simulink model "RechtenMotor_2_4_simu"  (R2012b)
settings: Solver=FixedStepDiscrete  StartTime=0.0  StopTime=10.0  RelTol=1e-3
undefined symbols (not defined in the file): sigbuilder_block
libraries: c2833xlib x1, c280xlib x1
settings Model: Creator=mit064  LastModifiedBy=Gelin Wang
settings DataIOCC: SaveOutput=off  SaveTime=off
settings OptimizationCC: OptimizeModelRefInitCode=on  LifeSpan=1
settings HardwareCC: ProdBitPerChar=16  ProdBitPerInt=16  ProdBitPerPointer=16  ProdLargestAtomicInteger=Integer  ProdIntDivRoundTo=Zero  ProdEndianess=LittleEndian  ProdWordSize=16  ProdHWDeviceType=Texas Instruments->C2000
settings RTWCC: SystemTargetFile=idelink_ert.tlc  GenerateMakefile=off  TemplateMakefile=none  Description=IDE Link ERT  ProcessScript=idelink_ert_make_rtw_hook
settings CodeAppCC: IgnoreCustomStorageClasses=off

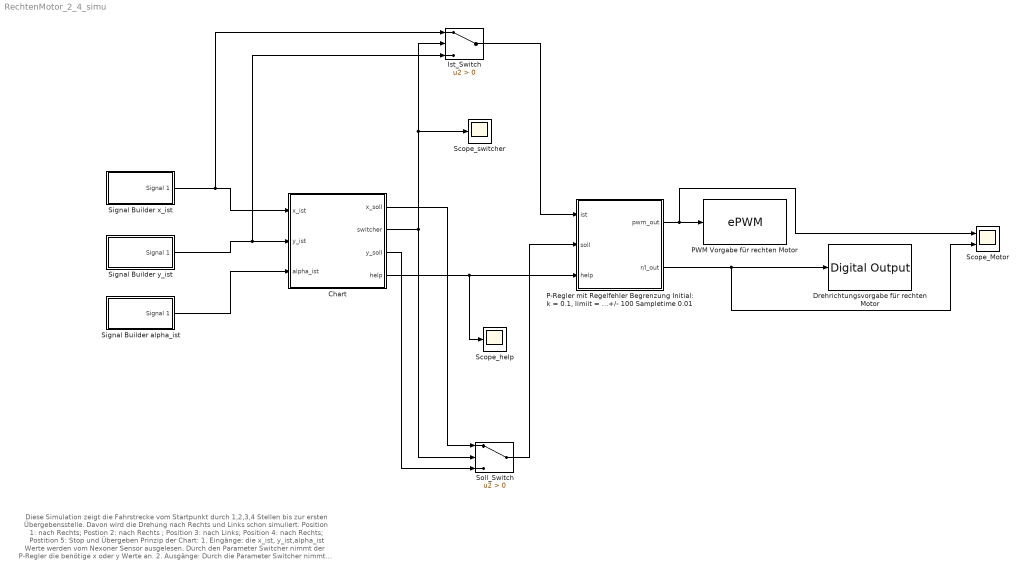
== system RechtenMotor_2_4_simu ==
  note: Diese Simulation zeigt die Fahrstrecke vom Startpunkt durch 1,2,3,4 Stellen bis zur ersten Übergebensstelle.
      | Davon wird die Drehung nach Rechts und Links schon simuliert.
      | Position 1: nach Rechts; Postion 2: nach Rechts ; Position 3: nach Links; Position 4: nach Rechts; Postition 5: Stop und Übergeben
      |
      | Prinzip der Chart:
      | 1. Eingänge: die x_ist, y_ist,alpha_ist Werte werden vom Nexoner Sensor ausgelesen.
      | Durch den Parameter Switcher nimmt der P-Regler die benötige x oder y Werte an.
      | 2. Ausgänge: Durch die Parameter Switcher nimmt ebenfalls der P-Regler die benötige x oder y Werte an.
      | 3. Parameter help in Ausgang: im Fall wenn der Fahrzeug sich nach Rechts umdrehen will, und  y_soll oder x_soll werte kleiner als den letzen Stelle ist,
      | wird "help" gleich eins, somit dreht sich der Rechtsmotor in negative Richtung .
      | 4. Parameter help in P-Regler: wenn help gleich eins ist, wird der Motor sich  immer in eine Richtung drehen.
  Chart : Stateflow chart  TreatAsAtomicUnit=on
  Drehrichtungsvorgabe für rechten Motor : c2833xlib/Digital Output  GPIO_Number=GPIO16~GPIO23  GPIO_Bit0=off  GPIO_BIT0_Toggle=off  GPIO_Bit1=off  GPIO_BIT1_Toggle=off  GPIO_Bit2=off  GPIO_BIT2_Toggle=off  GPIO_Bit3=off  GPIO_BIT3_Toggle=off  GPIO_Bit4=off  GPIO_BIT4_Toggle=off  GPIO_Bit5=on  GPIO_BIT5_Toggle=off  GPIO_Bit6=off  GPIO_BIT6_Toggle=off  GPIO_Bit7=off  GPIO_BIT7_Toggle=off
  Ist_Switch : Switch  Criteria=u2 > Threshold
  "P-Regler mit Regelfehler Begrenzung Initial: k = 0.1, limiit = +/- 100 Sampletime 0.01" : Subsystem
  "PWM Vorgabe für rechten Motor " : c280xlib/ePWM  checkMode=off  useModule=ePWM2  periodUnits=Clock cycles  timerSource=Specify via dialog  timerPeriod_clk=64000  timerPeriod_sec=0.0001  countingMode=Up  synchronizationOption=Disable  synchronizationEnable=off  phaseActiveEnable=Disable  phaseDirection=Count down after sync  phaseActive=0  clockPrescale=1  HSclockPrescale=1  ePWMxAStatus=off  CMPAUnits=Clock cycles  CMPASource=Specify via dialog  CMPAValue_per=50  CMPAValue_clk=32000  ePWMxAactionLogic1=Do nothing  ePWMxAactionLogic2=Clear  ePWMxAactionLogic3=Set  ePWMxAactionLogic4=Do nothing  ePWMxAactionLogic5=Do nothing  ePWMxAactionLogic6=Do nothing  ePWMxALoadMode=Load on CTR=Zero  ePWMxACSFenable=off  ePWMxACSFvalue=Forcing Disable  ePWMxASFreload=Zero  enHRPWM=off  HRPWM_LoadMode=CTR=ZERO  HRPWM_CTLMode=Phase control mode  HRPWM_EDGMode=Both edge  enSFO=on  ePWMxBStatus=on  CMPBUnits=Percentages  CMPBSource=Input port  CMPBValue_per=0  CMPBValue_clk=32000  ePWMxBactionLogic1=Do nothing  ePWMxBactionLogic2=Set  ePWMxBactionLogic3=Do nothing  ePWMxBactionLogic4=Do nothing  ePWMxBactionLogic5=Clear  ePWMxBactionLogic6=Do nothing  ePWMxBLoadMode=Load on CTR=Zero  ePWMxBCSFenable=off  ePWMxBCSFvalue=Forcing Disable  ePWMxBSFreload=Zero  enableDBePWMxA=off  enableDBePWMxB=off  DBpolarity=AH  DBedgeDelay=Positive  DBSource_ePWMxA=ePWMxA  DBSource_ePWMxB=ePWMxA  DBperiodSource=Specify via dialog  REDperiod=0  FEDperiod=0  adcstartModuleA=off  adcrequestEventA=First event  adcstartEventA=CTR=Zero  adcstartModuleB=off  adcrequestEventB=First event  adcstartEventB=CTR=Zero  intEn=off  intPrd=First event  intSel=CTR=Zero  chopperEnable=off  chopperFrequency=1  chopperFirstwidth=1  chopperDuty=12.5%  tripZonesource=Specify via dialog  tzselOSHT1=off  tzselOSHT2=off  tzselOSHT3=off  tzselOSHT4=off  tzselOSHT5=off  tzselOSHT6=off  tzselCBC1=off  tzselCBC2=off  tzselCBC3=off  tzselCBC4=off  tzselCBC5=off  tzselCBC6=off  enTzOstIntr=off  enTzCbcIntr=off  ePWMxAforced=No action  ePWMxBforced=No action  timerPeriod=-1  ePWMxAValue=0  ePWMxBValue=0  tripZoneoption=OSHT
  Scope_Motor : Scope  NumInputPorts=2
      settings: YMin=-5~-5  YMax=120~5
  Scope_help : Scope
      settings: SaveName=ScopeData2
  "Scope_switcher " : Scope
  "Signal Builder alpha_ist " : Subsystem  Tag=STV Subsys  LoadFcn=sigbuilder_block('load');  StartFcn=sigbuilder_block('start');  StopFcn=sigbuilder_block('stop');  ClipboardFcn=sigbuilder_block('clipboard');  mask(Sigbuilder block){}
      mask help: Simulink:masks:SigbuilderBlock_MD
      mask init:
      | if ~strcmp(get_param(bdroot(gcbh),'SimulationStatus'),'stopped') tuvar = sigbuilder_block('maskInit'); end
      settings: CopyFcn=sigbuilder_block('copy');  DeleteFcn=sigbuilder_block('delete');  ModelCloseFcn=sigbuilder_block('modelClose');  PreSaveFcn=sigbuilder_block('preSave');  PauseFcn=sigbuilder_block('pause');  ContinueFcn=sigbuilder_block('continue');  NameChangeFcn=sigbuilder_block('namechange');  OpenFcn=sigbuilder_block('open',[803.25 -542.25 550.5 399.75 ]);  CloseFcn=sigbuilder_block('close');
      mask Display: plot(0, 0, 100, 100,[2, 2, 32, 32, 2], [68, 8, 8, 68, 68],[32, 2], [38, 38], [32, 19, 2],[53, 60, 44], [32, 17, 17, 2],[16, 16, 31, 31]);txt = getActiveGroup(gcbh);text(2, 100, txt,'verticalAlignment', 'top');
  "Signal Builder x_ist " : Subsystem  Tag=STV Subsys  LoadFcn=sigbuilder_block('load');  StartFcn=sigbuilder_block('start');  StopFcn=sigbuilder_block('stop');  ClipboardFcn=sigbuilder_block('clipboard');  mask(Sigbuilder block){}
      mask help: Simulink:masks:SigbuilderBlock_MD
      mask init:
      | if ~strcmp(get_param(bdroot(gcbh),'SimulationStatus'),'stopped') tuvar = sigbuilder_block('maskInit'); end
      settings: CopyFcn=sigbuilder_block('copy');  DeleteFcn=sigbuilder_block('delete');  ModelCloseFcn=sigbuilder_block('modelClose');  PreSaveFcn=sigbuilder_block('preSave');  PauseFcn=sigbuilder_block('pause');  ContinueFcn=sigbuilder_block('continue');  NameChangeFcn=sigbuilder_block('namechange');  OpenFcn=sigbuilder_block('open',[403.5 2.25 550.5 399.75 ]);  CloseFcn=sigbuilder_block('close');
      mask Display: plot(0, 0, 100, 100,[2, 2, 32, 32, 2], [68, 8, 8, 68, 68],[32, 2], [38, 38], [32, 19, 2],[53, 60, 44], [32, 17, 17, 2],[16, 16, 31, 31]);txt = getActiveGroup(gcbh);text(2, 100, txt,'verticalAlignment', 'top');
  "Signal Builder y_ist " : Subsystem  Tag=STV Subsys  LoadFcn=sigbuilder_block('load');  StartFcn=sigbuilder_block('start');  StopFcn=sigbuilder_block('stop');  ClipboardFcn=sigbuilder_block('clipboard');  mask(Sigbuilder block){}
      mask help: Simulink:masks:SigbuilderBlock_MD
      mask init:
      | if ~strcmp(get_param(bdroot(gcbh),'SimulationStatus'),'stopped') tuvar = sigbuilder_block('maskInit'); end
      settings: CopyFcn=sigbuilder_block('copy');  DeleteFcn=sigbuilder_block('delete');  ModelCloseFcn=sigbuilder_block('modelClose');  PreSaveFcn=sigbuilder_block('preSave');  PauseFcn=sigbuilder_block('pause');  ContinueFcn=sigbuilder_block('continue');  NameChangeFcn=sigbuilder_block('namechange');  OpenFcn=sigbuilder_block('open',[1200.75 -1.5 550.5 399.75 ]);  CloseFcn=sigbuilder_block('close');
      mask Display: plot(0, 0, 100, 100,[2, 2, 32, 32, 2], [68, 8, 8, 68, 68],[32, 2], [38, 38], [32, 19, 2],[53, 60, 44], [32, 17, 17, 2],[16, 16, 31, 31]);txt = getActiveGroup(gcbh);text(2, 100, txt,'verticalAlignment', 'top');
  Soll_Switch : Switch  Criteria=u2 > Threshold
  wires:
  "P-Regler mit Regelfehler Begrenzung Initial: k = 0.1, limiit = +/- 100 Sampletime 0.01"/2(r/l_out) -> Scope_Motor/2, Drehrichtungsvorgabe für rechten Motor/1
  "P-Regler mit Regelfehler Begrenzung Initial: k = 0.1, limiit = +/- 100 Sampletime 0.01"/1(pwm_out) -> Scope_Motor/1, "PWM Vorgabe für rechten Motor "/1
  Ist_Switch/1 -> "P-Regler mit Regelfehler Begrenzung Initial: k = 0.1, limiit = +/- 100 Sampletime 0.01"/1(ist)
  Soll_Switch/1 -> "P-Regler mit Regelfehler Begrenzung Initial: k = 0.1, limiit = +/- 100 Sampletime 0.01"/2(soll)
  Chart/2(switcher) -> "Scope_switcher "/1, Ist_Switch/2, Soll_Switch/2
  Chart/1(x_soll) -> Soll_Switch/1
  Chart/3(y_soll) -> Soll_Switch/3
  Chart/4(help) -> Scope_help/1, "P-Regler mit Regelfehler Begrenzung Initial: k = 0.1, limiit = +/- 100 Sampletime 0.01"/3(help)
  "Signal Builder x_ist "/1(Signal 1) -> Ist_Switch/1, Chart/1(x_ist)
  "Signal Builder y_ist "/1(Signal 1) -> Ist_Switch/3, Chart/2(y_ist)
  "Signal Builder alpha_ist "/1(Signal 1) -> Chart/3(alpha_ist)

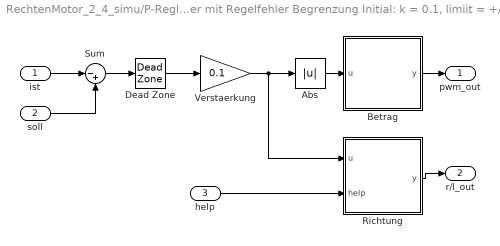
== system RechtenMotor_2_4_simu/P-Regler mit Regelfehler Begrenzung Initial: k = 0.1, limiit = +//- 100 Sampletime 0.01 ==
  ist : Inport
  soll : Inport  Port=2
  help : Inport  Port=3
  Abs : Abs  SampleTime=0.01
  Betrag : MATLAB Function  TreatAsAtomicUnit=on  SystemSampleTime=0.01
  Dead Zone : DeadZone  LowerValue=-100  UpperValue=100  SampleTime=0.01  SaturateOnIntegerOverflow=on
  Richtung : MATLAB Function  TreatAsAtomicUnit=on  SystemSampleTime=0.01
  Sum : Sum  Inputs=|-+  SampleTime=0.01
  Verstaerkung : Gain  Gain=0.1  SampleTime=0.01
  pwm_out : Outport
  r/l_out : Outport  Port=2
  wires:
  Betrag/1(y) -> pwm_out/1
  Sum/1 -> Dead Zone/1
  Verstaerkung/1 -> Abs/1, Richtung/1(u)
  Dead Zone/1 -> Verstaerkung/1
  Abs/1 -> Betrag/1(u)
  soll/1 -> Sum/2
  Richtung/1(y) -> r/l_out/1
  ist/1 -> Sum/1
  help/1 -> Richtung/2(help)

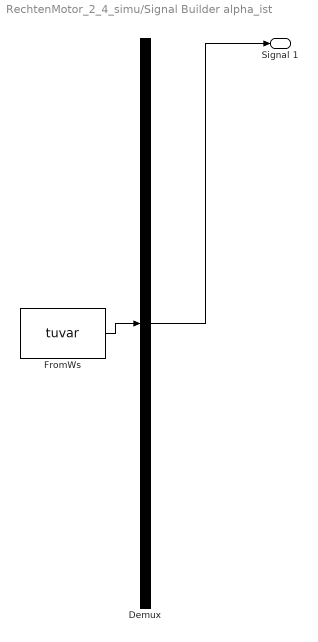
== system RechtenMotor_2_4_simu/Signal Builder alpha_ist  ==
  Demux : Demux  Tag=STV Demux  Outputs=1
  FromWs : FromWorkspace  Tag=STV FromWs  VariableName=tuvar  SampleTime=0
      SigBuilderData=|
      | common.afterFinalStr = 'Extrapolate'
      | common.sampleTime = 0
      | dataSet.timeRange = [0 25]
      | dataSet.name = 'Group 1'
      | sbobj.Groups.Name = 'Group 1'
      | sbobj.Groups.Signals.Name = 'Signal 1'
      | sbobj.Groups.Signals.XData = [0 4 5 6 9.5 10.5 14 15 18.5 19.5 25]
      | sbobj.Groups.Signals.YData = [90 90 90 77 77 -59 -59 63 63 -63 -63]
      | sbobj.Groups.TimeRange = [0 25]
  Signal 1 : Outport  Tag=STV Outport
  wires:
  Demux/1 -> Signal 1/1
  FromWs/1 -> Demux/1

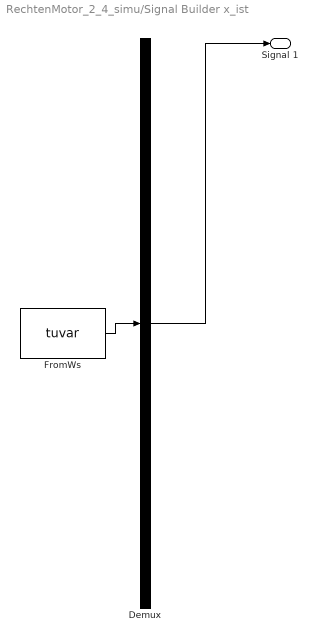
== system RechtenMotor_2_4_simu/Signal Builder x_ist  ==
  Demux : Demux  Tag=STV Demux  Outputs=1
  FromWs : FromWorkspace  Tag=STV FromWs  VariableName=tuvar  SampleTime=0
      SigBuilderData=|
      | common.afterFinalStr = 'Extrapolate'
      | common.sampleTime = 0
      | dataSet.timeRange = [0 25]
      | dataSet.name = 'Group 1'
      | sbobj.Groups.Name = 'Group 1'
      | sbobj.Groups.Signals.Name = 'Signal 1'
      | sbobj.Groups.Signals.XData = [0 4 6 6.5 8.5 11 13 15.5 17.5 20 22 25]
      | sbobj.Groups.Signals.YData = [350 350 350 350 500 500 800 800 950 950 1100 1100]
      | sbobj.Groups.TimeRange = [0 25]
  Signal 1 : Outport  Tag=STV Outport
  wires:
  Demux/1 -> Signal 1/1
  FromWs/1 -> Demux/1

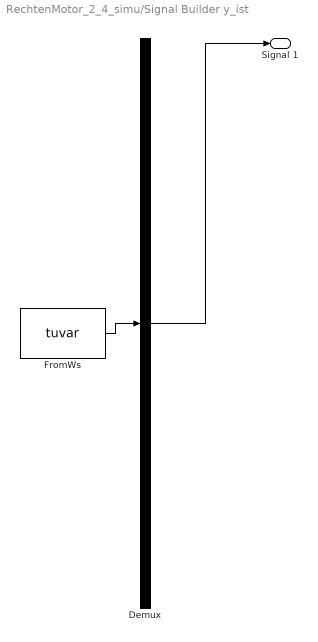
== system RechtenMotor_2_4_simu/Signal Builder y_ist  ==
  Demux : Demux  Tag=STV Demux  Outputs=1
  FromWs : FromWorkspace  Tag=STV FromWs  VariableName=tuvar  SampleTime=0
      SigBuilderData=|
      | common.afterFinalStr = 'Extrapolate'
      | common.sampleTime = 0
      | dataSet.timeRange = [0 25]
      | dataSet.name = 'Group 1'
      | sbobj.Groups.Name = 'Group 1'
      | sbobj.Groups.Signals.Name = 'Signal 1'
      | sbobj.Groups.Signals.XData = [0 2 4 6 6.5 8.5 11 13 15.5 17.5 20 22 25]
      | sbobj.Groups.Signals.YData = [0 0 250 250 250 900 900 400 400 700 700 400 400]
      | sbobj.Groups.TimeRange = [0 25]
  Signal 1 : Outport  Tag=STV Outport
  wires:
  Demux/1 -> Signal 1/1
  FromWs/1 -> Demux/1

== stateflow chart RechtenMotor_2_4_simu/Chart ==
  state Start
  state Position_3
    exit:switcher=0;
    exit:help=1;
    state Position_2
      entry:y_soll=400;
    state Stop
      entry:y_soll=y_ist;
    state Drehen_Linke
      entry:y_soll=0;
    state stop
      entry:y_soll=y_ist;
    (default) -> Position_3.Position_2
    Position_3.Position_2 -> Position_3.Stop : [y_ist<402&&y_ist>398]
    Position_3.Stop -> Position_3.Drehen_Linke : [after(1,sec)]
    Position_3.Drehen_Linke -> Position_3.stop : [alpha_ist<65&&alpha_ist>61]
  state Position_4
    exit:switcher=0;
    exit:help=0;
    state Position_3
      entry:y_soll=700;
    state Stop
      entry:y_soll=y_ist;
    state Drehen_Recht
      entry:y_soll=0;
    state stop
      entry:y_soll=y_ist;
    (default) -> Position_4.Position_3
    Position_4.Position_3 -> Position_4.Stop : [y_ist<702&&y_ist>698]
    Position_4.Stop -> Position_4.Drehen_Recht : [after(1,sec)]
    Position_4.Drehen_Recht -> Position_4.stop : [alpha_ist<-61&&alpha_ist>-65]
  state Position_1
    exit:switcher=0;
    exit:help=0;
    state Position_1
      entry:y_soll=350;
    state Stop
      entry:y_soll=y_ist;
    state Drehen_Recht
      entry:y_soll=0;
    state stop
      entry:y_soll=y_ist;
    (default) -> Position_1.Position_1
    Position_1.Position_1 -> Position_1.Stop : [y_ist<352&&y_ist>348]
    Position_1.Stop -> Position_1.Drehen_Recht : [after(1,sec)]
    Position_1.Drehen_Recht -> Position_1.stop : [alpha_ist<79&&alpha_ist>75]
  state Position_2
    exit:switcher=0;
    exit:help=0;
    state Position_2
      entry:y_soll=900;
    state Stop
      entry:y_soll=y_ist;
    state Drehen_Recht
      entry:y_soll=0;
    state stop
      entry:y_soll=y_ist;
    (default) -> Position_2.Position_2
    Position_2.Position_2 -> Position_2.Stop : [y_ist<902&&y_ist>898]
    Position_2.Stop -> Position_2.Drehen_Recht : [after(1,sec)]
    Position_2.Drehen_Recht -> Position_2.stop : [alpha_ist>-61&&alpha_ist<-57]
  state Position_6
    exit:switcher=0;
    exit:help=1;
    state Position_2
      entry:y_soll=300;
    state Stop
      entry:y_soll=y_ist;
    state Drehen_Linke
      entry:y_soll=0;
    state stop
      entry:y_soll=y_ist;
    (default) -> Position_6.Position_2
    Position_6.Position_2 -> Position_6.Stop : [y_ist<302&&y_ist>298]
    Position_6.Stop -> Position_6.Drehen_Linke : [after(1,sec)]
    Position_6.Drehen_Linke -> Position_6.stop : [alpha_ist<-32&&alpha_ist>-36]
  state Position_5_give
    exit:switcher=0;
    exit:help=0;
    state Position_1
      entry:y_soll=400;
    state Stop
      entry:y_soll=y_ist;
    state Drehen_Recht
      entry:y_soll=0;
    state stop
      entry:y_soll=y_ist;
    (default) -> Position_5_give.Position_1
    Position_5_give.Position_1 -> Position_5_give.Stop : [y_ist<402&&y_ist>398]
    Position_5_give.Stop -> Position_5_give.Drehen_Recht : [after(5,sec)]
    Position_5_give.Drehen_Recht -> Position_5_give.stop : [alpha_ist<-88]
  state Position_7
    exit:switcher=1;
    exit:help=1;
    state Position_2
      entry:x_soll=1400;
    state Stop
      entry:x_soll=x_ist;
    state Drehen_Linke
      entry:x_soll=0;
    state stop
      entry:x_soll=x_ist;
    (default) -> Position_7.Position_2
    Position_7.Position_2 -> Position_7.Stop : [x_ist<1402&&x_ist>1398]
    Position_7.Stop -> Position_7.Drehen_Linke : [after(1,sec)]
    Position_7.Drehen_Linke -> Position_7.stop : [alpha_ist<47&&alpha_ist>43]
  state Position_8
    exit:switcher=1;
    exit:help=1;
    state Position_2
      entry:x_soll=1700;
    state Stop
      entry:x_soll=x_ist;
    state Drehen_Linke
      entry:x_soll=0;
    state stop
      entry:x_soll=x_ist;
    (default) -> Position_8.Position_2
    Position_8.Position_2 -> Position_8.Stop : [x_ist<1702&&x_ist>1698]
    Position_8.Stop -> Position_8.Drehen_Linke : [after(1,sec)]
    Position_8.Drehen_Linke -> Position_8.stop : [alpha_ist<47&&alpha_ist>43]
  state Position_11_give
    exit:switcher=0;
    exit:help=1;
    state Position_2
      entry:y_soll=300;
    state Stop
      entry:y_soll=y_ist;
    (default) -> Position_11_give.Position_2
    Position_11_give.Position_2 -> Position_11_give.Stop : [y_ist<302&&y_ist>298]
  state Position_12_End
    exit:switcher=0;
    exit:help=1;
    state Position_2
      entry:y_soll=-200;
    state Stop
      entry:y_soll=y_ist;
    (default) -> Position_12_End.Position_2
    Position_12_End.Position_2 -> Position_12_End.Stop : [y_ist<-198&&y_ist>-202]
  state Position_9
    exit:switcher=1;
    exit:help=1;
    state Position_2
      entry:x_soll=1100;
    state Stop
      entry:x_soll=x_ist;
    state Drehen_Linke
      entry:x_soll=0;
    state stop
      entry:x_soll=x_ist;
    (default) -> Position_9.Position_2
    Position_9.Position_2 -> Position_9.Stop : [x_ist<1102&&x_ist>1098]
    Position_9.Stop -> Position_9.Drehen_Linke : [after(1,sec)]
    Position_9.Drehen_Linke -> Position_9.stop : [alpha_ist<2&&alpha_ist>-2]
  state Position_10
    exit:switcher=0;
    exit:help=1;
    state Position_2
      entry:y_soll=300;
    state Stop
      entry:y_soll=y_ist;
    state Drehen_Linke
      entry:y_soll=0;
    state stop
      entry:y_soll=y_ist;
    (default) -> Position_10.Position_2
    Position_10.Position_2 -> Position_10.Stop : [y_ist<302&&y_ist>298]
    Position_10.Stop -> Position_10.Drehen_Linke : [after(1,sec)]
    Position_10.Drehen_Linke -> Position_10.stop : [alpha_ist<-88]
  (default) -> Start
  Start -> Position_1 : [after(2,sec)]
  Position_3 -> Position_4 : [after(0.5,sec)]
  Position_1 -> Position_2 : [after(0.5,sec)]
  Position_2 -> Position_3 : [after(0.5,sec)]
  Position_4 -> Position_5_give : [after(0.5,sec)]
  Position_7 -> Position_8 : [after(0.5,sec)]
  Position_6 -> Position_7 : [after(0.5,sec)]
  Position_5_give -> Position_6 : [after(0.5,sec)]
  Position_8 -> Position_9 : [after(0.5,sec)]
  Position_11_give -> Position_12_End : [after(5,sec)]
  Position_9 -> Position_10 : [after(0.5,sec)]
  Position_10 -> Position_11_give : [after(0.5,sec)]
  data: x_ist input; y_ist input; alpha_ist input; x_soll output; switcher output; y_soll output; help output

== matlab function RechtenMotor_2_4_simu/P-Regler mit Regelfehler Begrenzung Initial: k = 0.1, limiit = +//- 100 Sampletime 0.01/Betrag ==
  settings: updateMethod=DISCRETE  sampleTime=0.01
  data: u input; y output
function y = fcn( u )

if 0.5 < u && u < 60
    y = 60;
elseif u <= 0.5
    y = 0;
elseif u >= 100
    y = 100;
else
    y = abs(u);
end

== matlab function RechtenMotor_2_4_simu/P-Regler mit Regelfehler Begrenzung Initial: k = 0.1, limiit = +//- 100 Sampletime 0.01/Richtung ==
  settings: updateMethod=DISCRETE  sampleTime=0.01
  data: u input; y output; help input
function y = fcn( u,help) 

if u > 0
    y = 1;
else
    y = 0+help;
end
